simulink model "pendulum"  (R2021b)
settings: Solver=VariableStepAuto  StartTime=0.0  StopTime=30.0  MaxStep=0.01  RelTol=1e-3
libraries: simulink_extras x1
settings Model: Creator=user  LastModifiedBy=user

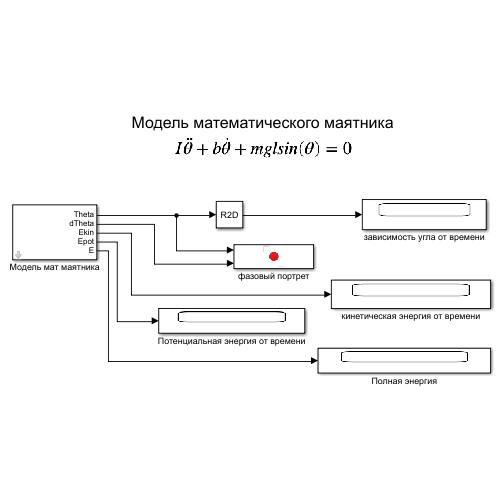
[thumbnail: Simulink's stored preview of the top-level diagram]
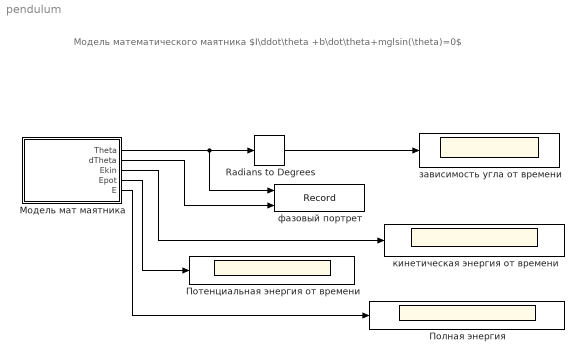
== system pendulum ==
  note: Модель математического маятника
      | $I\ddot\theta +b\dot\theta+mglsin(\theta)=0$
  Radians to Degrees : simulink_extras/Transformations/Radians to Degrees
  Модель мат маятника : Subsystem  mask{m=1, l=1, g=9.81, startDegree=30, b=0.2}
      mask prompts: m "Масса"; l "Длина подвеса"; g "Ускорение свободного падения"; startDegree "Стартовый угол"; b "Коэффициент затухания"
      mask init:
      | I = m*l*l
  Полная энергия : Scope
  Потенциальная энергия от времени : Scope
  зависимость угла от времени : Scope
  кинетическая энергия от времени : Scope
  фазовый портрет : Record  FileSettingsInternal="{\"entries\":[{\"content\":{\"excelSettings\":{\"content\":{},\"type\":\"Streamout.ExcelSettings\"}},\"type\":\"Streamout.FileSettingStorage\",\"uuid\":\"06ce8ab5-a378-48c7-8448-b12ee1caa920\"}],\"packageUris\":[\"http://schema.mathworks.com/mf0/streamout_blocks/R2020a\"],\"version\":\"1.0\"}"  Layout=[1 1]  SignalsInternal="{\"entries\":[{\"content\":{\"signals\":[{\"content\":{\"blockPath\":[\"pendulum/фазовый портрет\"],\"channel\":[],\"dimensions\":[1],\"domain\":\"pendulum/￯﾿ﾽ￯﾿ﾽ￯﾿ﾽ￯﾿ﾽ￯﾿ﾽ￯﾿ﾽ￯﾿ﾽ ￯﾿ﾽ￯﾿ﾽ￯﾿ﾽ￯﾿ﾽ￯﾿ﾽ￯﾿ﾽ￯﾿ﾽ\",\"lineColor\":\"#77ac30\",\"plots\":[],\"port\":1,\"sid\":[\"\"],\"signalID\":414,\"signalName\":\"Модель мат маятника:1\"},\"type\":\"RecordBlkView.Signal\",\"uuid\":\"16637b75-59d9-4aa1-a3c6-adcbd7455cd1\"},{\"content\":{\"blockPath\":[\"pendulum/фазовый портрет\"],\"channel\":[],\"dimensions\":[1],\"domain\":\"pendulum/￯﾿ﾽ￯﾿ﾽ￯﾿ﾽ￯﾿ﾽ￯﾿ﾽ￯﾿ﾽ￯﾿ﾽ ￯﾿ﾽ￯﾿ﾽ￯﾿ﾽ￯﾿ﾽ￯﾿ﾽ￯﾿ﾽ￯﾿ﾽ\",\"lineColor\":\"#4dbeee\",\"plots\":[],\"port\":2,\"sid\":[\"\"],\"signalID\":418,\"signalName\":\"Модель мат маятника:2\"},\"type\":\"RecordBlkView.Signal\",\"uuid\":\"ef2761da-8680-48f5-b183-b662f56edb9e\"}]},\"type\":\"RecordBlkView.InputSignals\",\"uuid\":\"e5e70cc5-7c7e-4f97-a1aa-71d20f42ea56\"}],\"packageUris\":[\"http://schema.mathworks.com/mf0/streamout_blocks/R2020a\"],\"version\":\"1.0\"}"  VisualizationBindings="{\"xyplotplugin\":{\"info\":[{\"series\":[],\"subplotID\":1}]}}"  CompatibilityTag=XY
  wires:
  Radians to Degrees/1 -> зависимость угла от времени/1
  Модель мат маятника/1(Theta) -> фазовый портрет/1, Radians to Degrees/1
  Модель мат маятника/2(dTheta) -> фазовый портрет/2
  Модель мат маятника/4(Epot) -> Потенциальная энергия от времени/1
  Модель мат маятника/3(Ekin) -> кинетическая энергия от времени/1
  Модель мат маятника/5(E) -> Полная энергия/1

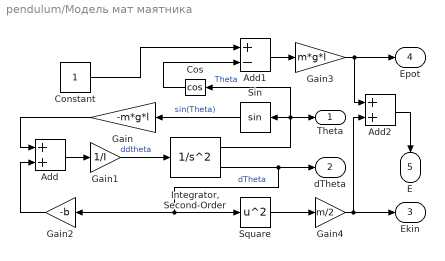
== system pendulum/Модель мат маятника ==
  Add : Sum
  Add1 : Sum  Inputs=+-
  Add2 : Sum
  Constant : Constant
  Cos : Trigonometry  Operator=cos
  Gain : Gain  Gain=-m*g*l
  Gain1 : Gain  Gain=1/I
  Gain2 : Gain  Gain=-b
  Gain3 : Gain  Gain=m*g*l
  Gain4 : Gain  Gain=m/2
  "Integrator, Second-Order" : SecondOrderIntegrator  ICX=deg2rad(startDegree)
  Sin : Trigonometry
  Square : Math  Operator=square  SaturateOnIntegerOverflow=on
  Theta : Outport
  dTheta : Outport  Port=2
  Ekin : Outport  Port=3
  Epot : Outport  Port=4
  E : Outport  Port=5
  wires:
  "Integrator, Second-Order"/1 -> Theta/1, Cos/1, Sin/1  "Theta"
  Gain1/1 -> "Integrator, Second-Order"/1  "ddtheta"
  Sin/1 -> Gain/1  "sin(Theta)"
  Gain/1 -> Add/1
  Add/1 -> Gain1/1
  "Integrator, Second-Order"/2 -> Gain2/1, Square/1, dTheta/1  "dTheta"
  Gain2/1 -> Add/2
  Cos/1 -> Add1/2
  Constant/1 -> Add1/1
  Gain3/1 -> Add2/1, Epot/1
  Add1/1 -> Gain3/1
  Square/1 -> Gain4/1
  Gain4/1 -> Add2/2, Ekin/1
  Add2/1 -> E/1
